simulink model "MultiPortSwitch_4"  (R2017b)
settings: Solver=FixedStepDiscrete  StartTime=0.0  StopTime=10.0  FixedStep=0.200000  RelTol=1e-3
settings Model: Creator=hbourbou  LastModifiedBy=hbourbou
settings DataIOCC: SaveFormat=StructureWithTime
settings OptimizationCC: LifeSpan=inf
settings DebuggingCC: SFExecutionAtInitializationDiag=none
settings HardwareCC: ProdBitPerSizeT=32  ProdBitPerPtrDiffT=32  ProdWordSize=32  ProdHWDeviceType=Specified
settings CodeAppCC: StateflowObjectComments=on

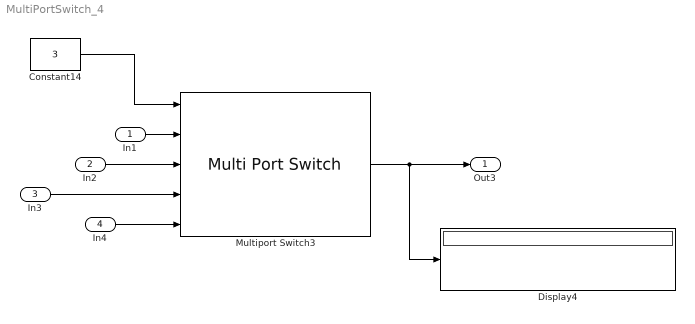
== system MultiPortSwitch_4 ==
  In1 : Inport  PortDimensions=[2,3]
  In2 : Inport  Port=2  PortDimensions=[2,3]
  In3 : Inport  Port=3  PortDimensions=[2,3]
  In4 : Inport  Port=4  PortDimensions=[2,3]
  Constant14 : Constant  Value=3
  Display4 : Display
  Multiport Switch3 : MultiPortSwitch  DataPortForDefault=Additional data port
  Out3 : Outport
  wires:
  Constant14/1 -> Multiport Switch3/1
  Multiport Switch3/1 -> Display4/1, Out3/1
  In1/1 -> Multiport Switch3/2
  In2/1 -> Multiport Switch3/3
  In3/1 -> Multiport Switch3/4
  In4/1 -> Multiport Switch3/5
